simulink model "motor_LA_NDr"  (R2023b)
settings: Solver=FixedStepAuto  StartTime=0.0  StopTime=3  RelTol=1e-3  EnableMultiTasking=on
libraries: mbedblockslib x6, simulink x1
settings Model: SimulationMode=external  ExtModeTrigDuration=10  Creator=damia  LastModifiedBy=Usuario
settings SolverCC: AlgebraicLoopSolver=TrustRegion
settings OptimizationCC: EnhancedBackFolding=on  PassReuseOutputArgsThreshold=0  MaxStackSize=64  SimCompilerOptimization=on  OptimizeBlockOrder=speed  DifferentSizesBufferReuse=on  OptimizationCustomize=off
settings DebuggingCC: ParameterTunabilityLossMsg=error  UnconnectedInputMsg=warning  UnconnectedOutputMsg=warning  UnconnectedLineMsg=warning
settings HardwareCC: ProdBitPerPointer=32  ProdBitPerSizeT=32  ProdBitPerPtrDiffT=32  ProdLargestAtomicInteger=Long  ProdLargestAtomicFloat=Double  ProdWordSize=32  ProdHWDeviceType=ARM Compatible->ARM Cortex  UseEmbeddedCoderFeatures=off
settings ModelReferenceCC: EnableRefExpFcnMdlSchedulingChecks=on
settings SFSimCC: MATLABDynamicMemAlloc=off  CustomCodeUndefinedFunction=UseInterfaceOnly
settings RTWCC: Description=Embedded Coder  SystemTargetFile=ert.tlc  HardwareBoard=STM32 Nucleo F411RE  TemplateMakefile=ert_default_tmf  GenerateReport=on  Toolchain=GNU Tools for ARM Embedded Processors  LaunchReport=on  DLArmComputeVersion=19.05
settings CodeAppCC: ForceParamTrailComments=on  OperatorAnnotations=on
settings ERTTargetCC: ERTCustomFileBanners=off  SupportContinuousTime=on  SupportNonInlinedSFcns=on  RemoveResetFunc=off  ModelStepFunctionPrototypeControlCompliant=off  ExtModeTransport=3  ExtModeStaticAlloc=on  ExtModeStaticAllocSize=2000  ExtModeMexFile=ext_xcp  ExtModeIntrfLevel=Level2 - Open

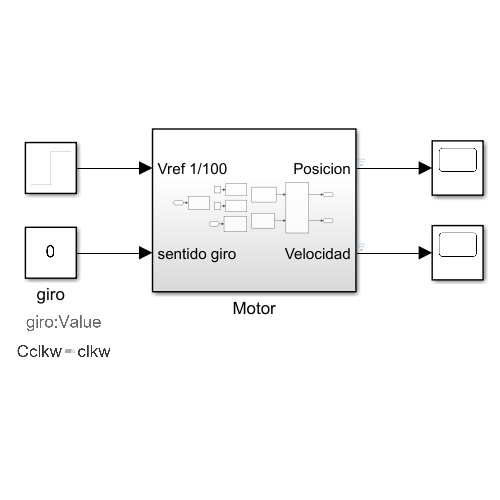
[thumbnail: Simulink's stored preview of the top-level diagram]
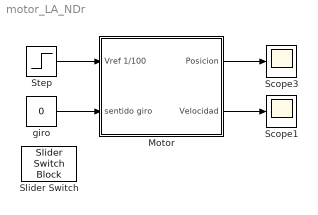
== system motor_LA_NDr ==
  Motor : Subsystem
  Scope1 : Scope
  Scope3 : Scope
  Slider Switch : SliderSwitchBlock
      settings: Values={{'Cclkw', 'clkw'}, [1 0]}
  Step : Step  Time=0  After=50  SampleTime=0.0001
  giro : Constant  Value=0
  wires:
  Motor/1(Posicion) -> Scope3/1
  Motor/2(Velocidad) -> Scope1/1
  Step/1 -> Motor/1(Vref 1/100)
  giro/1 -> Motor/2(sentido giro)

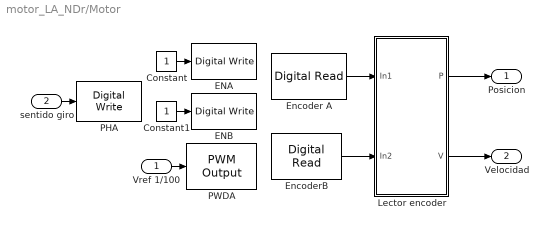
== system motor_LA_NDr/Motor ==
  Vref 1/100 : Inport
  sentido giro : Inport  Port=2
  Constant : Constant
  Constant1 : Constant
  ENA : mbedblockslib/Digital Write  Pin=D2  Direction=output
  ENB : mbedblockslib/Digital Write  Pin=D11  Direction=output
  Encoder A : mbedblockslib/Digital Read  Pin=A1  Direction=input  SampleTime=0.0001
  EncoderB : mbedblockslib/Digital Read  Pin=A0  Direction=input  SampleTime=0.0001
  Lector encoder : Subsystem
  PHA : mbedblockslib/Digital Write  Pin=D3  Direction=output
  PWDA : mbedblockslib/PWM Output  Pin=D5  EnableInputFrequency=off  InitialFrequency=5000  InitialDutyCycle=50  NotificationType=None
  Posicion : Outport  VectorParamsAs1DForOutWhenUnconnected=off
  Velocidad : Outport  Port=2  VectorParamsAs1DForOutWhenUnconnected=off
  wires:
  Encoder A/1 -> Lector encoder/1(In1)
  EncoderB/1 -> Lector encoder/2(In2)
  Lector encoder/2(V) -> Velocidad/1
  Lector encoder/1(P) -> Posicion/1
  Constant/1 -> ENA/1
  Constant1/1 -> ENB/1
  Vref 1/100/1 -> PWDA/1
  sentido giro/1 -> PHA/1

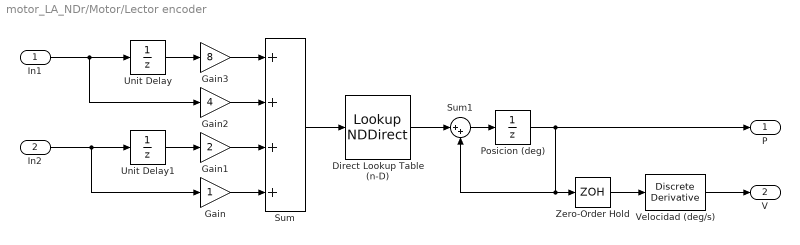
== system motor_LA_NDr/Motor/Lector encoder ==
  In1 : Inport
  In2 : Inport  Port=2
  Direct Lookup Table (n-D) : LookupNDDirect  NumberOfTableDimensions=1  Table=[0,-1,1,0,1,0,0,-1,-1,0,0,1,0,1,-1,0]
  Gain : Gain
  Gain1 : Gain  Gain=2
  Gain2 : Gain  Gain=4
  Gain3 : Gain  Gain=8
  Posicion (deg) : UnitDelay  SampleTime=-1  HasFrameUpgradeWarning=on
  Sum : Sum  Inputs=++++  OutDataTypeStr=double
  Sum1 : Sum  Inputs=|++
  Unit Delay : UnitDelay  SampleTime=-1  HasFrameUpgradeWarning=on
  Unit Delay1 : UnitDelay  SampleTime=-1  HasFrameUpgradeWarning=on
  Velocidad (deg/s) : simulink/Discrete/Discrete Derivative  gainval=1  ICPrevScaledInput=0.0  OutMin=[]  OutMax=[]  OutDataType=fixdt(1, 16)  OutScaling=2^-10  DoSatur=off
  Zero-Order Hold : ZeroOrderHold  SampleTime=0.01
  P : Outport  VectorParamsAs1DForOutWhenUnconnected=off
  V : Outport  Port=2  VectorParamsAs1DForOutWhenUnconnected=off
  wires:
  Sum1/1 -> Posicion (deg)/1
  In2/1 -> Gain/1, Unit Delay1/1
  Posicion (deg)/1 -> Sum1/2, Zero-Order Hold/1, P/1
  Unit Delay1/1 -> Gain1/1
  In1/1 -> Unit Delay/1, Gain2/1
  Gain1/1 -> Sum/3
  Gain/1 -> Sum/4
  Gain3/1 -> Sum/1
  Gain2/1 -> Sum/2
  Unit Delay/1 -> Gain3/1
  Zero-Order Hold/1 -> Velocidad (deg/s)/1
  Velocidad (deg/s)/1 -> V/1
  Sum/1 -> Direct Lookup Table (n-D)/1
  Direct Lookup Table (n-D)/1 -> Sum1/1
